simulink model "task_2"  (R2023b)
settings: Solver=FixedStepAuto  StartTime=0.0  StopTime=50  FixedStep=1e-3  RelTol=1e-3
values from neighbouring files (symbols this model uses):
  A = [0, 1; -a0 -a1] + [0 0; 20 20]    [task_2.m]    (also in task_3.m)
  A_M = [0 1; -a_M0 -a_M1]    [task_2.m]    (also in task_3.m)
  b = [0; b0]    [task_2.m]    (also in task_3.m)
  b_M = [0; a_M0]    [task_2.m]    (also in task_3.m)
  C = eye(2)    [task_2.m]    (also in task_3.m)
  kappa = b0/a_M0    (= 0.074549499703)    [task_2.m]    (also in task_3.m)
settings Model: Creator=nguye  LastModifiedBy=nguye

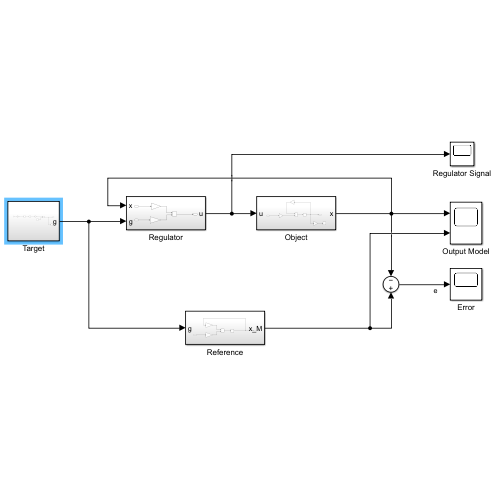
[thumbnail: Simulink's stored preview of the top-level diagram]
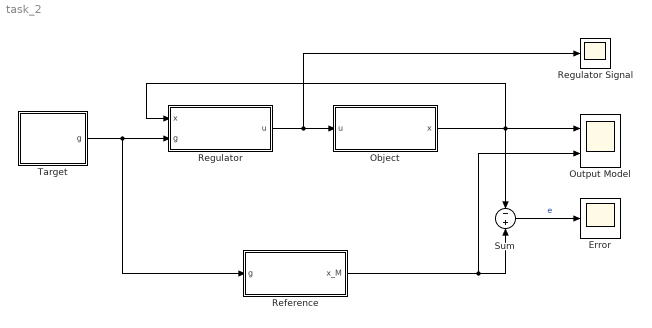
== system task_2 ==
  Error : Scope
  Object : Subsystem
  Output Model : Scope  NumInputPorts=2
  Reference : Subsystem
  Regulator : Subsystem
  Regulator Signal : Scope
  Sum : Sum  Inputs=-|+
  Target : Subsystem
  wires:
  Target/1(g) -> Regulator/2(g), Reference/1(g)
  Sum/1 -> Error/1  "e"
  Regulator/1(u) -> Regulator Signal/1, Object/1(u)
  Reference/1(x_M) -> Output Model/2, Sum/2
  Object/1(x) -> Output Model/1, Regulator/1(x), Sum/1

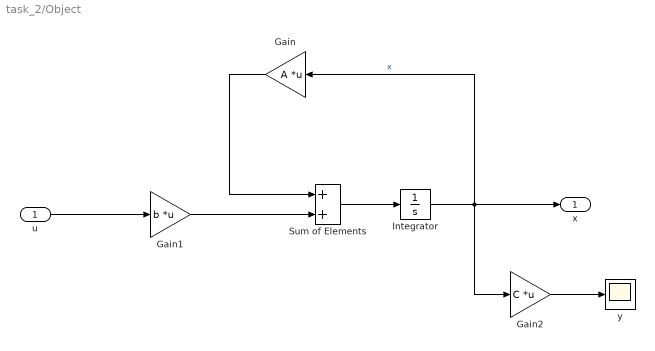
== system task_2/Object ==
  u : Inport
  Gain : Gain  Gain=A  Multiplication=Matrix(K*u)
  Gain1 : Gain  Gain=b  Multiplication=Matrix(K*u)
  Gain2 : Gain  Gain=C  Multiplication=Matrix(K*u)
  Integrator : Integrator  InitialCondition=1
  Sum of Elements : Sum
  y : Scope
  x : Outport
  wires:
  Sum of Elements/1 -> Integrator/1
  Gain/1 -> Sum of Elements/1
  Gain1/1 -> Sum of Elements/2
  u/1 -> Gain1/1
  Integrator/1 -> Gain/1, Gain2/1, x/1  "x"
  Gain2/1 -> y/1

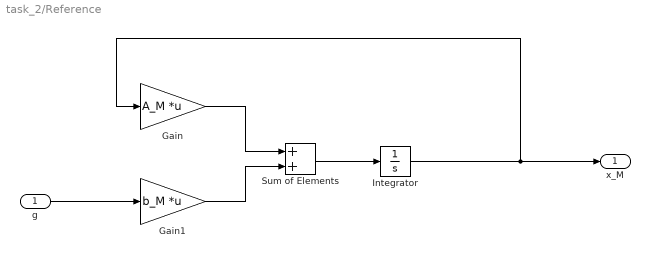
== system task_2/Reference ==
  g : Inport
  Gain : Gain  Gain=A_M  Multiplication=Matrix(K*u)
  Gain1 : Gain  Gain=b_M  Multiplication=Matrix(K*u)
  Integrator : Integrator
  Sum of Elements : Sum
  x_M : Outport
  wires:
  g/1 -> Gain1/1
  Gain1/1 -> Sum of Elements/2
  Gain/1 -> Sum of Elements/1
  Sum of Elements/1 -> Integrator/1
  Integrator/1 -> Gain/1, x_M/1

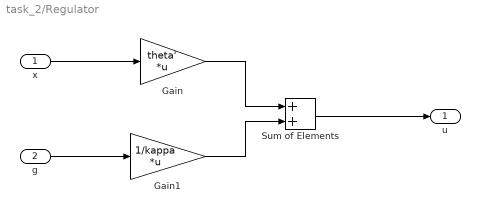
== system task_2/Regulator ==
  x : Inport
  g : Inport  Port=2
  Gain : Gain  Gain=theta'  Multiplication=Matrix(K*u)
  Gain1 : Gain  Gain=1/kappa  Multiplication=Matrix(K*u)
  Sum of Elements : Sum
  u : Outport
  wires:
  x/1 -> Gain/1
  Gain/1 -> Sum of Elements/1
  Gain1/1 -> Sum of Elements/2
  g/1 -> Gain1/1
  Sum of Elements/1 -> u/1

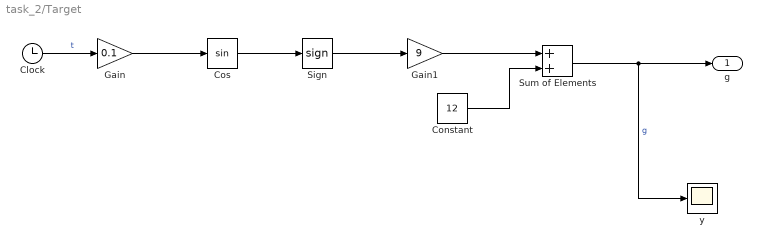
== system task_2/Target ==
  Clock : Clock
  Constant : Constant  Value=12
  Cos : Trigonometry
  Gain : Gain  Gain=0.1
  Gain1 : Gain  Gain=9
  Sign : Signum
  Sum of Elements : Sum
  y : Scope
  g : Outport
  wires:
  Clock/1 -> Gain/1  "t"
  Cos/1 -> Sign/1
  Sign/1 -> Gain1/1
  Constant/1 -> Sum of Elements/2
  Sum of Elements/1 -> y/1, g/1  "g"
  Gain/1 -> Cos/1
  Gain1/1 -> Sum of Elements/1
